simulink library "Autonomous_lib"  (R2023b)
settings: Solver=VariableStepAuto  StartTime=0.0  StopTime=10.0  RelTol=1e-3
undefined symbols (not defined in the file): Spline_Num_Poses_default, Spline_Ref_Poses_default
settings Model: Creator=FIRSTMentor  LastModifiedBy=ander

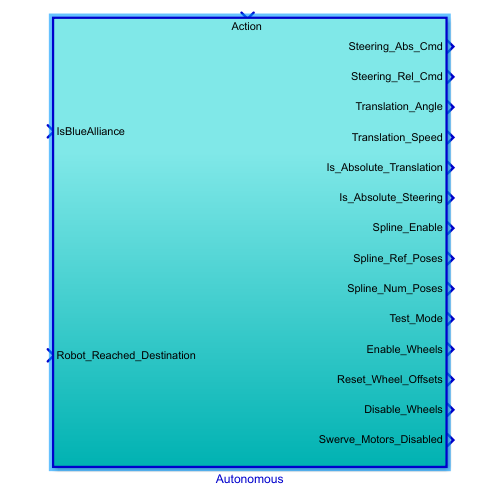
[thumbnail: Simulink's stored preview of the top-level diagram]
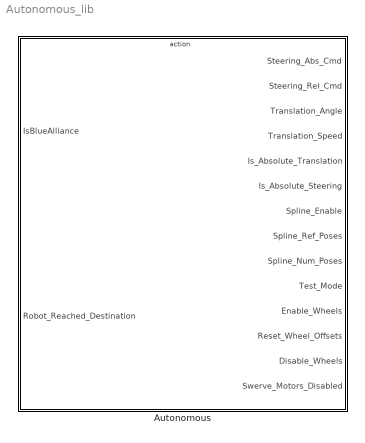
== system Autonomous_lib ==
  Autonomous : Subsystem  TreatAsAtomicUnit=on

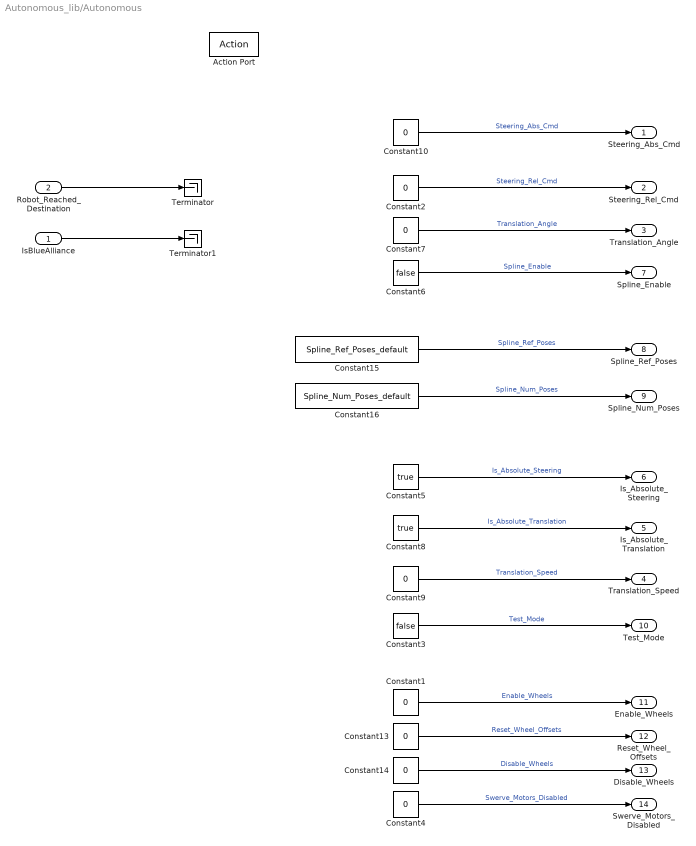
== system Autonomous_lib/Autonomous ==
  IsBlueAlliance : Inport
  Robot_Reached_Destination : Inport  Port=2
  Action Port : ActionPort  InitializeStates=reset
  Constant{1..2,7,9..10,13..14} (7 alike) : Constant  Value=0
  Constant15 : Constant  Value=Spline_Ref_Poses_default
  Constant16 : Constant  Value=Spline_Num_Poses_default  OutDataTypeStr=double
  Constant3 : Constant  Value=false  OutDataTypeStr=boolean
  Constant4 : Constant  Value=0  OutDataTypeStr=boolean
  Constant5 : Constant  Value=true
  Constant6 : Constant  Value=false
  Constant8 : Constant  Value=true
  Terminator : Terminator
  Terminator1 : Terminator
  Steering_Abs_Cmd : Outport
  Steering_Rel_Cmd : Outport  Port=2
  Translation_Angle : Outport  Port=3
  Translation_Speed : Outport  Port=4
  Is_Absolute_Translation : Outport  Port=5
  Is_Absolute_Steering : Outport  Port=6
  Spline_Enable : Outport  Port=7
  Spline_Ref_Poses : Outport  Port=8
  Spline_Num_Poses : Outport  Port=9
  Test_Mode : Outport  Port=10
  Enable_Wheels : Outport  Port=11
  Reset_Wheel_Offsets : Outport  Port=12
  Disable_Wheels : Outport  Port=13
  Swerve_Motors_Disabled : Outport  Port=14
  wires:
  Constant2/1 -> Steering_Rel_Cmd/1  "Steering_Rel_Cmd"
  Constant15/1 -> Spline_Ref_Poses/1  "Spline_Ref_Poses"
  Constant7/1 -> Translation_Angle/1  "Translation_Angle"
  Constant3/1 -> Test_Mode/1  "Test_Mode"
  Constant14/1 -> Disable_Wheels/1  "Disable_Wheels"
  Constant13/1 -> Reset_Wheel_Offsets/1  "Reset_Wheel_Offsets"
  Constant4/1 -> Swerve_Motors_Disabled/1  "Swerve_Motors_Disabled"
  Constant1/1 -> Enable_Wheels/1  "Enable_Wheels"
  Robot_Reached_Destination/1 -> Terminator/1
  IsBlueAlliance/1 -> Terminator1/1
  Constant5/1 -> Is_Absolute_Steering/1  "Is_Absolute_Steering"
  Constant8/1 -> Is_Absolute_Translation/1  "Is_Absolute_Translation"
  Constant9/1 -> Translation_Speed/1  "Translation_Speed"
  Constant6/1 -> Spline_Enable/1  "Spline_Enable"
  Constant10/1 -> Steering_Abs_Cmd/1  "Steering_Abs_Cmd"
  Constant16/1 -> Spline_Num_Poses/1  "Spline_Num_Poses"
